simulink model "pendulo"  (Simulink 9.1)
settings: Solver=ode45  StartTime=0.0  StopTime=30  RelTol=1e-3  EnableMultiTasking=on
values from neighbouring files (symbols this model uses):
  b = 0.5    [main.m]
  g = 9.81    [main.m]
  L = 1.5    [main.m]
settings Model: Creator=oscar  LastModifiedBy=oscar
settings DataIOCC: LimitDataPoints=on  Refine=10
settings DebuggingCC: UnderspecifiedInitializationDetection=Simplified  MergeDetectMultiDrivingBlocksExec=error  SolverPrmCheckMsg=warning
settings GRTTargetCC: GeneratePreprocessorConditionals=Disable all  CombineOutputUpdateFcns=on  GRTInterface=off
settings ConfigComp: CovSFcnEnable=off
settings SimscapeCC: SimscapeNormalizeSystem=off
settings ConfigurationSet: Description=SimMechanics 2G

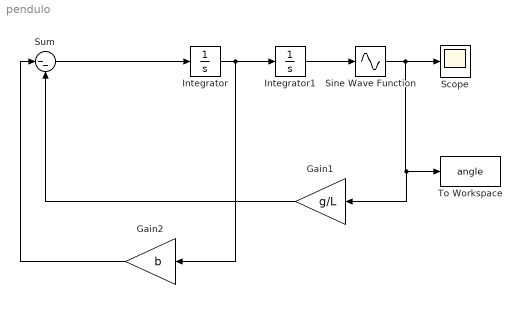
== system pendulo ==
  Gain1 : Gain  Gain=g/L
  Gain2 : Gain  Gain=b
  Integrator : Integrator
  Integrator1 : Integrator  InitialCondition=0.5
  Scope : Scope
  Sine Wave Function : Sin  TimeSource=Use external signal  SampleTime=0
  Sum : Sum  Inputs=|--
  To Workspace : ToWorkspace  VariableName=angle  SaveFormat=Timeseries  SampleTime=-1
  wires:
  Integrator/1 -> Gain2/1, Integrator1/1
  Sum/1 -> Integrator/1
  Integrator1/1 -> Sine Wave Function/1
  Sine Wave Function/1 -> Scope/1, Gain1/1, To Workspace/1
  Gain1/1 -> Sum/2
  Gain2/1 -> Sum/1
